simulink model "hand_dryer_controller_R2022B"  (R2022b)
settings: Solver=FixedStepDiscrete  StartTime=0.0  StopTime=100  FixedStep=0.1  RelTol=1e-3
PostLoadFcn:
  | run("DesiredSolverSetting.m");
settings Model: Creator=ACER  LastModifiedBy=ACER
settings OptimizationCC: DefaultParameterBehavior=Inlined  ReuseModelBlockBuffer=on  EnhancedBackFolding=on  PassReuseOutputArgsAs=Individual arguments  ZeroExternalMemoryAtStartup=off  ZeroInternalMemoryAtStartup=off  OptimizeBlockOrder=speed  DifferentSizesBufferReuse=on  OptimizationCustomize=off  EfficientTunableParamExpr=on
settings DebuggingCC: ParameterTunabilityLossMsg=error
settings SFSimCC: MATLABDynamicMemAlloc=off
settings RTWCC: Description=Embedded Coder  SystemTargetFile=ert.tlc  GenCodeOnly=on  TemplateMakefile=ert_default_tmf  GPUComputeCapability=5.0
settings CodeAppCC: ForceParamTrailComments=on  IgnoreCustomStorageClasses=off  OperatorAnnotations=on  SimulinkDataObjDesc=on  SFDataObjDesc=on  InsertBlockDesc=on
settings ERTTargetCC: TargetLangStandard=C99 (ISO)  GenerateSampleERTMain=on  InlinedParameterPlacement=NonHierarchical  ERTCustomFileTemplate=example_file_process.tlc
settings ConfigComp: CovEnable=on  RecordCoverage=on  CovMetricSettings=dcmwe  CovModelRefEnable=on

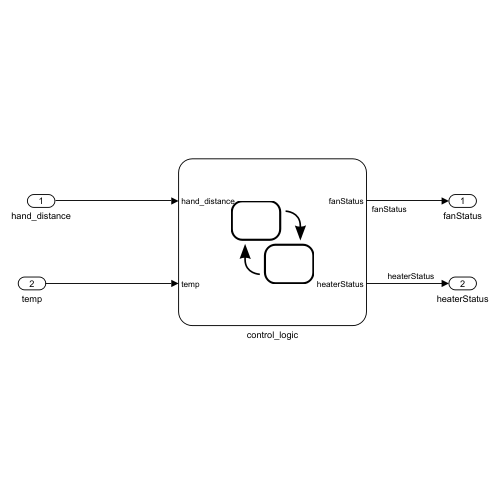
[thumbnail: Simulink's stored preview of the top-level diagram]
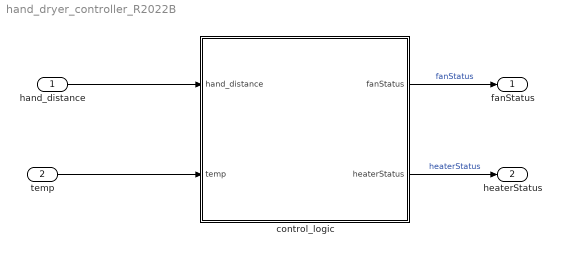
== system hand_dryer_controller_R2022B ==
  hand_distance : Inport
  temp : Inport  Port=2
  control_logic : Stateflow chart  TreatAsAtomicUnit=on
  fanStatus : Outport
  heaterStatus : Outport  Port=2
  wires:
  control_logic/1(fanStatus) -> fanStatus/1  "fanStatus"
  hand_distance/1 -> control_logic/1(hand_distance)
  control_logic/2(heaterStatus) -> heaterStatus/1  "heaterStatus"
  temp/1 -> control_logic/2(temp)

== stateflow chart hand_dryer_controller_R2022B/control_logic ==
  state Idle
    en:
    fanStatus = Off;
    heaterStatus = Off;
  state Active
    state lowTemp
      en:
      fanStatus=On;
      heaterStatus = On;
    state highTemp
      en:
      fanStatus = On;
      heaterStatus = Off;
    (default) -> (junction 52)
    (junction 52) -> highTemp [order 2]
    (junction 52) -> lowTemp [order 1] : [temp<65]
    highTemp -> lowTemp : [temp<65]
    lowTemp -> highTemp : [temp>=70]
  state waitState
  state waiteState2
  (default) -> Idle
  Idle -> waitState : [hand_distance<10]
  waitState -> Active [order 2] : after(1,sec)
  waitState -> Idle [order 1] : [hand_distance>=10]
  Active -> waiteState2 [order 1] : [hand_distance>15]
  waiteState2 -> Active [order 1] : [hand_distance<=15]
  waiteState2 -> Idle [order 2] : after(3,sec)
  Active -> Idle [order 2] : after(60,sec)
  data: hand_distance input; temp input; fanStatus output Enum: OnOffEnum; heaterStatus output Enum: OnOffEnum
